simulink model "tumblingOnly"  (R2020a)
settings: Solver=ode8  StartTime=0.0  StopTime=observationTime  FixedStep=timeStep  RelTol=1e-3
values from neighbouring files (symbols this model uses):
  ICStructure = getICStructure(SpacecraftStructure.J_transverse, SpacecraftStructure.J_z, MU)    [runDocking.m]
undefined symbols (not defined in the file or in its folder): CT_BI0, initialConditionSet, wT_B0
libraries: TBMPC_Blocks x1
settings Model: Creator=hough  LastModifiedBy=hough

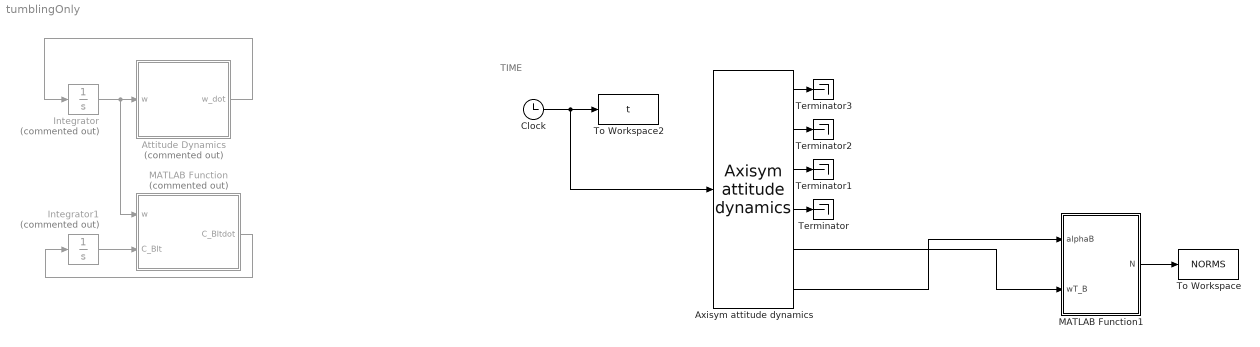
== system tumblingOnly ==
  note: TIME
  Attitude Dynamics : MATLAB Function  Commented=on  TreatAsAtomicUnit=on
  Axisym attitude dynamics : TBMPC_Blocks/Axisym attitude dynamics  J_transverse=SpacecraftStructure.J_transverse  J_z=SpacecraftStructure.J_z  omega_t=ICStructure.w_t{initialConditionSet}  omega_z=ICStructure.w_z{initialConditionSet}  mu_0=ICStructure.mu0{initialConditionSet}  gamma_0=ICStructure.gamma{initialConditionSet}  theta_0=ICStructure.theta0{initialConditionSet}
  Clock : Clock
  Integrator : Integrator  Commented=on  InitialCondition=wT_B0
  Integrator1 : Integrator  Commented=on  InitialCondition=CT_BI0
  MATLAB Function : MATLAB Function  Commented=on  TreatAsAtomicUnit=on
  MATLAB Function1 : MATLAB Function  TreatAsAtomicUnit=on
  Terminator{,1..3} (4 alike) : Terminator
  To Workspace : ToWorkspace  VariableName=NORMS  SampleTime=-1
  To Workspace2 : ToWorkspace  VariableName=t  SampleTime=-1
  wires:
  MATLAB Function/1(C_BItdot) -> Integrator1/1
  Integrator1/1 -> MATLAB Function/2(C_BIt)
  MATLAB Function1/1(N) -> To Workspace/1
  Clock/1 -> Axisym attitude dynamics/1, To Workspace2/1
  Integrator/1 -> MATLAB Function/1(w), Attitude Dynamics/1(w)
  Attitude Dynamics/1(w_dot) -> Integrator/1
  Axisym attitude dynamics/6 -> MATLAB Function1/1(alphaB)
  Axisym attitude dynamics/5 -> MATLAB Function1/2(wT_B)
  Axisym attitude dynamics/4 -> Terminator/1
  Axisym attitude dynamics/3 -> Terminator1/1
  Axisym attitude dynamics/2 -> Terminator2/1
  Axisym attitude dynamics/1 -> Terminator3/1

== matlab function tumblingOnly/MATLAB Function1 ==
  data: alphaB input; wT_B input; N output; d parameter
function N  = fcn(alphaB, wT_B, d)


N1 = norm((skew(wT_B)*skew(wT_B) + skew(alphaB))*d); % Acceleration of the docking cone
N2 = norm(skew(wT_B)*skew(wT_B) + skew(alphaB)); % For the r_D norm
N3 = norm(wT_B); % For the coriolis stuff


N = [N1;N2;N3];

== matlab function tumblingOnly/Attitude Dynamics ==
  data: w input; w_dot output; I parameter
function w_dot = fcn(w, I)

w_dot = -I\cross(w,I*w); % Changed from "inv" function to speed it up.

== matlab function tumblingOnly/MATLAB Function ==
  data: w input; C_BItdot output; C_BIt input
function C_BItdot = fcn(w,C_BIt)

w_skew = [0 -w(3) w(2)
          w(3) 0 -w(1)
          -w(2) w(1) 0];

C_BItdot = -w_skew*C_BIt;
